simulink model "BanlanceCar"  (R2021b)
settings: Solver=FixedStepDiscrete  StartTime=0.0  StopTime=10.0  MaxStep=0.001  RelTol=1e-3
libraries: TIMERS_Lib x11, GPIO_Lib x7, USART_Lib x3, REG_Lib x2, STM32_Config_Lib x1
settings Model: Creator=Daniel  LastModifiedBy=Daniel
settings OptimizationCC: DefaultParameterBehavior=Inlined  EnhancedBackFolding=on  PassReuseOutputArgsAs=Individual arguments  ZeroExternalMemoryAtStartup=off  ZeroInternalMemoryAtStartup=off  OptimizeBlockOrder=speed  DifferentSizesBufferReuse=on  OptimizationCustomize=off  EfficientTunableParamExpr=on
settings DebuggingCC: ParameterTunabilityLossMsg=error
settings SFSimCC: SimCustomHeaderCode="#include \"myfile.h\""  SimUserSources="\"D:\\Simulink_stm32f4\\STM32F407VET6\\BalanceCar\\myfile.c\""  MATLABDynamicMemAlloc=off  CustomCodeUndefinedFunction=UseInterfaceOnly
settings RTWCC: Description=stm32 (Embedded Target)  SystemTargetFile=stm32.tlc  TemplateMakefile=stm32.tmf  GenerateReport=on
settings CodeAppCC: ForceParamTrailComments=on  IgnoreCustomStorageClasses=off  MaxIdLength=64  OperatorAnnotations=on  SimulinkDataObjDesc=on  SFDataObjDesc=on  CustomSymbolStrType=$N$R$M  StateflowObjectComments=on  MATLABSourceComments=on
settings STFCustomTargetCC: TargetLangStandard=C99 (ISO)  CodeReplacementLibrary=ARM CMSIS SIN COS  MultiwordLength=256  ParMdlRefBuildCompliant=on  IncludeMdlTerminateFcn=off  CombineOutputUpdateFcns=on  ERTCustomFileBanners=on  SupportContinuousTime=off  SupportNonInlinedSFcns=off  RemoveResetFunc=on  MATLABClassNameForMDSCustomization=Simulink.SoftwareTarget.ERTCustomization  GRTInterface=off  SystemTargetFile=stm32.tlc
settings ERTTargetCC: TargetLangStandard=C99 (ISO)  CodeReplacementLibrary=ARM CMSIS SIN COS  CompOptLevelCompliant=off  ConcurrentExecutionCompliant=off  IncludeMdlTerminateFcn=off  ModelStepFunctionPrototypeControlCompliant=off  CPPClassGenCompliant=off  UseToolchainInfoCompliant=off  ExtModeStaticAllocSize=256  ExtModeMexFile=ext_serial_win32_comm  ExtModeMexArgs=0,1,115200,10  InlinedParameterPlacement=NonHierarchical  ERTSrcFileBannerTemplate=sourceFileTemplate.cgt  ERTHdrFileBannerTemplate=sourceFileTemplate.cgt  ERTDataSrcFileTemplate=sourceFileTemplate.cgt  ERTDataHdrFileTemplate=sourceFileTemplate.cgt  ERTCustomFileTemplate=customRoutineProcess.tlc

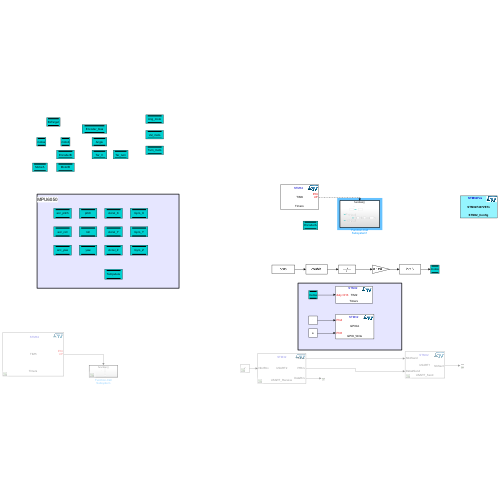
[thumbnail: Simulink's stored preview of the top-level diagram]
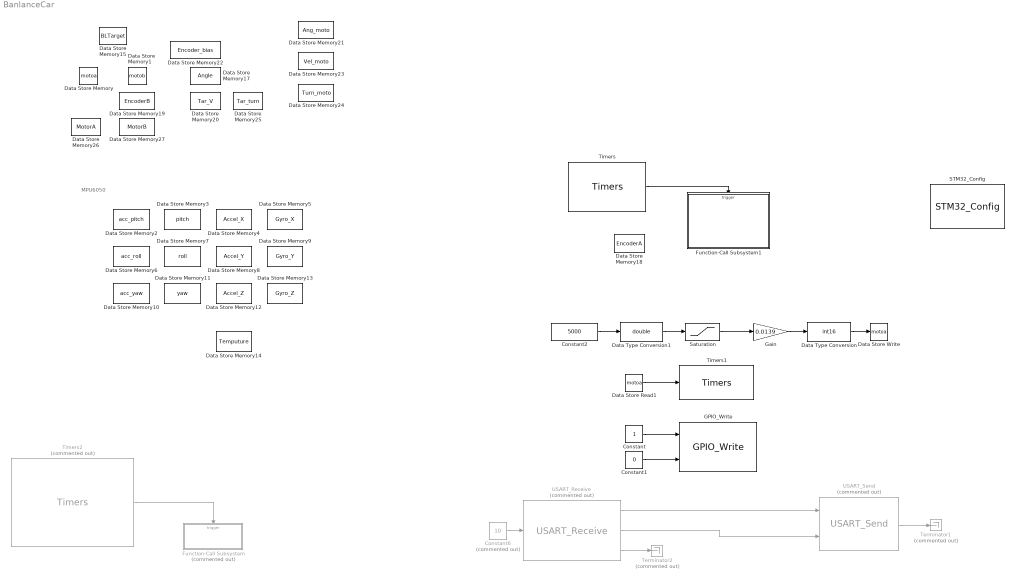
== system BanlanceCar ==
  note: MPU6050
  Constant : Constant
  Constant1 : Constant  Value=0
  Constant2 : Constant  Value=5000
  Constant6 : Constant  Commented=on  Value=10  OutDataTypeStr=uint16
  Data Store Memory : DataStoreMemory  DataStoreName=motoa  ReadBeforeWriteMsg=warning  WriteAfterWriteMsg=warning  WriteAfterReadMsg=warning  ShowAdditionalParam=off
  Data Store Memory1 : DataStoreMemory  DataStoreName=motob  ReadBeforeWriteMsg=warning  WriteAfterWriteMsg=warning  WriteAfterReadMsg=warning  ShowAdditionalParam=off
  Data Store Memory10 : DataStoreMemory  DataStoreName=acc_yaw  ReadBeforeWriteMsg=warning  WriteAfterWriteMsg=warning  WriteAfterReadMsg=warning  ShowAdditionalParam=off
  Data Store Memory11 : DataStoreMemory  DataStoreName=yaw  ReadBeforeWriteMsg=warning  WriteAfterWriteMsg=warning  WriteAfterReadMsg=warning  ShowAdditionalParam=off
  Data Store Memory12 : DataStoreMemory  DataStoreName=Accel_Z  ReadBeforeWriteMsg=warning  WriteAfterWriteMsg=warning  WriteAfterReadMsg=warning  ShowAdditionalParam=off
  Data Store Memory13 : DataStoreMemory  DataStoreName=Gyro_Z  ReadBeforeWriteMsg=warning  WriteAfterWriteMsg=warning  WriteAfterReadMsg=warning  ShowAdditionalParam=off
  Data Store Memory14 : DataStoreMemory  DataStoreName=Temputure  ReadBeforeWriteMsg=warning  WriteAfterWriteMsg=warning  WriteAfterReadMsg=warning  ShowAdditionalParam=off
  Data Store Memory15 : DataStoreMemory  DataStoreName=BLTarget  ReadBeforeWriteMsg=warning  WriteAfterWriteMsg=warning  WriteAfterReadMsg=warning  ShowAdditionalParam=off
  Data Store Memory17 : DataStoreMemory  DataStoreName=Angle  ReadBeforeWriteMsg=warning  WriteAfterWriteMsg=warning  WriteAfterReadMsg=warning  ShowAdditionalParam=off
  Data Store Memory18 : DataStoreMemory  DataStoreName=EncoderA  ReadBeforeWriteMsg=warning  WriteAfterWriteMsg=warning  WriteAfterReadMsg=warning  ShowAdditionalParam=off
  Data Store Memory19 : DataStoreMemory  DataStoreName=EncoderB  ReadBeforeWriteMsg=warning  WriteAfterWriteMsg=warning  WriteAfterReadMsg=warning  ShowAdditionalParam=off
  Data Store Memory2 : DataStoreMemory  DataStoreName=acc_pitch  ReadBeforeWriteMsg=warning  WriteAfterWriteMsg=warning  WriteAfterReadMsg=warning  ShowAdditionalParam=off
  Data Store Memory20 : DataStoreMemory  DataStoreName=Tar_V  ReadBeforeWriteMsg=warning  WriteAfterWriteMsg=warning  WriteAfterReadMsg=warning  ShowAdditionalParam=off
  Data Store Memory21 : DataStoreMemory  DataStoreName=Ang_moto  ReadBeforeWriteMsg=warning  WriteAfterWriteMsg=warning  WriteAfterReadMsg=warning  ShowAdditionalParam=off
  Data Store Memory22 : DataStoreMemory  DataStoreName=Encoder_bias  ReadBeforeWriteMsg=warning  WriteAfterWriteMsg=warning  WriteAfterReadMsg=warning  ShowAdditionalParam=off
  Data Store Memory23 : DataStoreMemory  DataStoreName=Vel_moto  ReadBeforeWriteMsg=warning  WriteAfterWriteMsg=warning  WriteAfterReadMsg=warning  ShowAdditionalParam=off
  Data Store Memory24 : DataStoreMemory  DataStoreName=Turn_moto  ReadBeforeWriteMsg=warning  WriteAfterWriteMsg=warning  WriteAfterReadMsg=warning  ShowAdditionalParam=off
  Data Store Memory25 : DataStoreMemory  DataStoreName=Tar_turn  ReadBeforeWriteMsg=warning  WriteAfterWriteMsg=warning  WriteAfterReadMsg=warning  ShowAdditionalParam=off
  Data Store Memory26 : DataStoreMemory  DataStoreName=MotorA  ReadBeforeWriteMsg=warning  WriteAfterWriteMsg=warning  WriteAfterReadMsg=warning  ShowAdditionalParam=off
  Data Store Memory27 : DataStoreMemory  DataStoreName=MotorB  ReadBeforeWriteMsg=warning  WriteAfterWriteMsg=warning  WriteAfterReadMsg=warning  ShowAdditionalParam=off
  Data Store Memory3 : DataStoreMemory  DataStoreName=pitch  ReadBeforeWriteMsg=warning  WriteAfterWriteMsg=warning  WriteAfterReadMsg=warning  ShowAdditionalParam=off
  Data Store Memory4 : DataStoreMemory  DataStoreName=Accel_X  ReadBeforeWriteMsg=warning  WriteAfterWriteMsg=warning  WriteAfterReadMsg=warning  ShowAdditionalParam=off
  Data Store Memory5 : DataStoreMemory  DataStoreName=Gyro_X  ReadBeforeWriteMsg=warning  WriteAfterWriteMsg=warning  WriteAfterReadMsg=warning  ShowAdditionalParam=off
  Data Store Memory6 : DataStoreMemory  DataStoreName=acc_roll  ReadBeforeWriteMsg=warning  WriteAfterWriteMsg=warning  WriteAfterReadMsg=warning  ShowAdditionalParam=off
  Data Store Memory7 : DataStoreMemory  DataStoreName=roll  ReadBeforeWriteMsg=warning  WriteAfterWriteMsg=warning  WriteAfterReadMsg=warning  ShowAdditionalParam=off
  Data Store Memory8 : DataStoreMemory  DataStoreName=Accel_Y  ReadBeforeWriteMsg=warning  WriteAfterWriteMsg=warning  WriteAfterReadMsg=warning  ShowAdditionalParam=off
  Data Store Memory9 : DataStoreMemory  DataStoreName=Gyro_Y  ReadBeforeWriteMsg=warning  WriteAfterWriteMsg=warning  WriteAfterReadMsg=warning  ShowAdditionalParam=off
  Data Store Read1 : DataStoreRead  DataStoreName=motoa  IndexOptions=Index vector (dialog)  Indices=1  OutputSizes=1
  Data Store Write : DataStoreWrite  DataStoreName=motoa  IndexOptions=Index vector (dialog)  Indices=1  OutputSizes=1
  Data Type Conversion : DataTypeConversion  OutDataTypeStr=int16
  Data Type Conversion1 : DataTypeConversion  OutDataTypeStr=double
  Function-Call Subsystem : Subsystem  Commented=on  TreatAsAtomicUnit=on
  Function-Call Subsystem1 : Subsystem  TreatAsAtomicUnit=on
  GPIO_Write : GPIO_Lib/GPIO_Write  Port_name=GPIOA  Pin0=off  Toggle_Pin0=off  Pin1=off  Toggle_Pin1=off  Pin2=off  Toggle_Pin2=off  Pin3=off  Toggle_Pin3=off  Pin4=on  Toggle_Pin4=off  Pin5=on  Toggle_Pin5=off  Pin6=off  Toggle_Pin6=off  Pin7=off  Toggle_Pin7=off  Pin8=off  Toggle_Pin8=off  Pin9=off  Toggle_Pin9=off  Pin10=off  Toggle_Pin10=off  Pin11=off  Toggle_Pin11=off  Pin12=off  Toggle_Pin12=off  Pin13=off  Toggle_Pin13=off  Pin14=off  Toggle_Pin14=off  Pin15=off  Toggle_Pin15=off  PinList="GPIOA4  5  6  7GPIOB9  10GPIOD1  2"
      settings: SourceProductName=Target Support Package - STM32 Adapter
  Gain : Gain  Gain=0.0139
  STM32_Config : STM32_Config_Lib/STM32_Config  Priority=0  Project_Path=.\  Config_File=BalanceCar.ioc  MCU_Name=STM32F407VETx
      settings: SourceProductName=Target Support Package - STM32 Adapter
  Saturation : Saturate  UpperLimit=7000  LowerLimit=-7000
  Terminator1 : Terminator  Commented=on
  Terminator2 : Terminator  Commented=on
  Timers : TIMERS_Lib/Timers  currentTIM=TIM9  TIM_Name=TIM9  sysUsingTimer=off  TIM_APBClock=72000000  TIM_Set_Clk=off  TIM_Prescaler=7199  TIM_Clock=10000.00  Variable_frequency=off  TIM_Set_OutFreq=off  TIM_ARR=10000  Output_frequency=1.00  Repetition_counter=0  TIM_Mode=Up  TIM_DMA=none  TIM_IRQ=on  TIM_IRQ_ONLY=on  TIM_UP=on  TIM_TRG=off  TIM_COM=off  TIM_BRK=off  NbTIM=5  CH1_enable=off  CH1N_enable=off  CH1_type=Unknown  CH1_DMA=off  CH1_int=off  CH1_edge=Rising  CH1_div=1  CH1_variable_duty=off  CH1_set_pulse=off  CH1_output_duty=0.00  CH1_pulse=0  CH2_enable=off  CH2N_enable=off  CH2_type=Unknown  CH2_DMA=off  CH2_int=off  CH2_edge=Rising  CH2_div=1  CH2_variable_duty=off  CH2_set_pulse=off  CH2_output_duty=0.00  CH2_pulse=0  CH3_enable=off  CH3N_enable=off  CH3_type=Unknown  CH3_DMA=off  CH3_int=off  CH3_edge=Rising  CH3_div=1  CH3_variable_duty=off  CH3_set_pulse=off  CH3_output_duty=0.00  CH3_pulse=0  CH4_enable=off  CH4N_enable=off  CH4_type=Unknown  CH4_DMA=off  CH4_int=off  CH4_edge=Rising  CH4_div=1  CH4_variable_duty=off  CH4_set_pulse=off  CH4_output_duty=0.00  CH4_pulse=0
      settings: SourceProductName=Target Support Package - STM32 Adapter
  Timers1 : TIMERS_Lib/Timers  currentTIM=TIM2  TIM_Name=TIM2  sysUsingTimer=off  TIM_APBClock=72000000  TIM_Set_Clk=off  TIM_Prescaler=0  TIM_Clock=72000000.00  Variable_frequency=off  TIM_Set_OutFreq=off  TIM_ARR=7199  Output_frequency=10001.39  Repetition_counter=0  TIM_Mode=Up  TIM_DMA=none  TIM_IRQ=on  TIM_IRQ_ONLY=off  TIM_UP=off  TIM_TRG=off  TIM_COM=off  TIM_BRK=off  NbTIM=5  CH1_enable=off  CH1N_enable=off  CH1_type=Unknown  CH1_DMA=off  CH1_int=off  CH1_edge=Rising  CH1_div=1  CH1_variable_duty=off  CH1_set_pulse=off  CH1_output_duty=0.00  CH1_pulse=0  CH2_enable=off  CH2N_enable=off  CH2_type=Unknown  CH2_DMA=off  CH2_int=off  CH2_edge=Rising  CH2_div=1  CH2_variable_duty=off  CH2_set_pulse=off  CH2_output_duty=0.00  CH2_pulse=0  CH3_enable=on  CH3N_enable=off  CH3_type=Output_PWM  CH3_DMA=off  CH3_int=off  CH3_edge=Rising  CH3_div=1  CH3_variable_duty=on  CH3_set_pulse=off  CH3_output_duty=6.93  CH3_pulse=500-1  CH4_enable=on  CH4N_enable=off  CH4_type=Output_PWM  CH4_DMA=off  CH4_int=off  CH4_edge=Rising  CH4_div=1  CH4_variable_duty=off  CH4_set_pulse=off  CH4_output_duty=0.00  CH4_pulse=0
      settings: SourceProductName=Target Support Package - STM32 Adapter
  Timers2 : TIMERS_Lib/Timers  Commented=on  currentTIM=TIM5  TIM_Name=TIM5  sysUsingTimer=off  TIM_APBClock=72000000  TIM_Set_Clk=off  TIM_Prescaler=7199  TIM_Clock=10000.00  Variable_frequency=off  TIM_Set_OutFreq=off  TIM_ARR=1  Output_frequency=10000.00  Repetition_counter=0  TIM_Mode=Up  TIM_DMA=none  TIM_IRQ=on  TIM_IRQ_ONLY=on  TIM_UP=on  TIM_TRG=off  TIM_COM=off  TIM_BRK=off  NbTIM=4  CH1_enable=off  CH1N_enable=off  CH1_type=Unknown  CH1_DMA=off  CH1_int=off  CH1_edge=Rising  CH1_div=1  CH1_variable_duty=off  CH1_set_pulse=off  CH1_output_duty=0.00  CH1_pulse=0  CH2_enable=off  CH2N_enable=off  CH2_type=Unknown  CH2_DMA=off  CH2_int=off  CH2_edge=Rising  CH2_div=1  CH2_variable_duty=off  CH2_set_pulse=off  CH2_output_duty=0.00  CH2_pulse=0  CH3_enable=off  CH3N_enable=off  CH3_type=Unknown  CH3_DMA=off  CH3_int=off  CH3_edge=Rising  CH3_div=1  CH3_variable_duty=off  CH3_set_pulse=off  CH3_output_duty=0.00  CH3_pulse=0  CH4_enable=off  CH4N_enable=off  CH4_type=Unknown  CH4_DMA=off  CH4_int=off  CH4_edge=Rising  CH4_div=1  CH4_variable_duty=off  CH4_set_pulse=off  CH4_output_duty=0.00  CH4_pulse=0
      settings: SourceProductName=Target Support Package - STM32 Adapter
  USART_Receive : USART_Lib/USART_Receive  Commented=on  USART_name=USART2  Buff_size=512  nbUsart=2  Soft_it=on  Soft_num=1  usartMode=Asynchronous  usartDma_Rx=off  usartDma_Tx=off  usartIt=on
      settings: SourceProductName=Target Support Package - STM32 Adapter
  USART_Send : USART_Lib/USART_Send  Commented=on  USART_name=USART1  Buff_size=512  nbUsart=2  usartMode=Asynchronous  usartDma_Rx=off  usartDma_Tx=off  usartIt=on
      settings: SourceProductName=Target Support Package - STM32 Adapter
  wires:
  USART_Receive/1 -> USART_Send/1
  Constant6/1 -> USART_Receive/1
  USART_Send/1 -> Terminator1/1
  USART_Receive/2 -> USART_Send/2
  USART_Receive/3 -> Terminator2/1
  Timers2/1 -> Function-Call Subsystem/Trigger
  Timers/1 -> Function-Call Subsystem1/Trigger
  Data Type Conversion1/1 -> Saturation/1
  Saturation/1 -> Gain/1
  Data Type Conversion/1 -> Data Store Write/1
  Gain/1 -> Data Type Conversion/1
  Constant1/1 -> GPIO_Write/2
  Constant/1 -> GPIO_Write/1
  Data Store Read1/1 -> Timers1/1
  Constant2/1 -> Data Type Conversion1/1

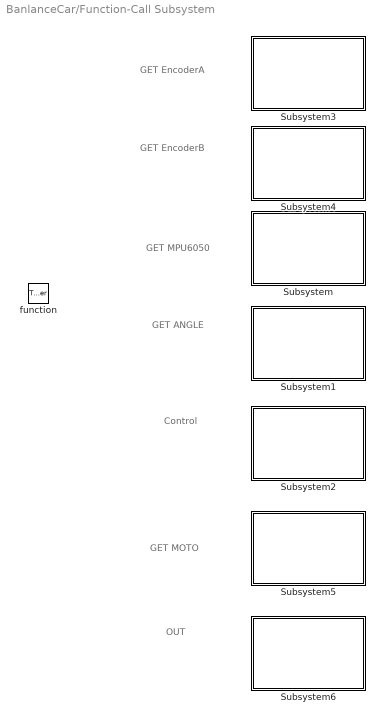
== system BanlanceCar/Function-Call Subsystem ==
  note: OUT
  note: GET MOTO
  note: GET EncoderB
  note: GET EncoderA
  note: Control
  note: GET ANGLE
  note: GET MPU6050
  function : TriggerPort  TriggerType=function-call  VariantControl=(inherit)
  Subsystem : Subsystem
  Subsystem1 : Subsystem
  Subsystem2 : Subsystem
  Subsystem3 : Subsystem
  Subsystem4 : Subsystem
  Subsystem5 : Subsystem
  Subsystem6 : Subsystem

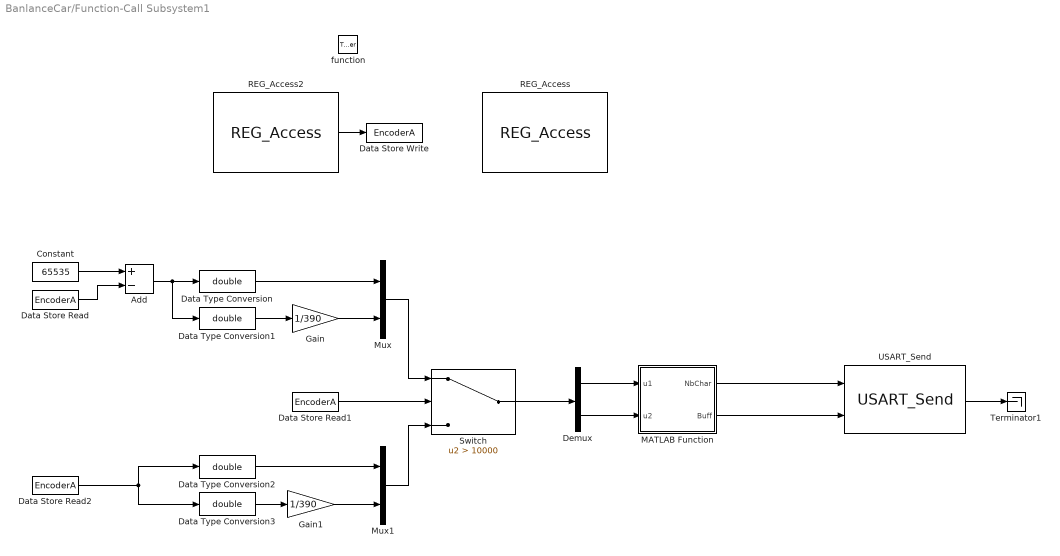
== system BanlanceCar/Function-Call Subsystem1 ==
  function : TriggerPort  TriggerType=function-call  VariantControl=(inherit)
  Add : Sum  Inputs=+-
  Constant : Constant  Value=65535
  Data Store Read : DataStoreRead  DataStoreName=EncoderA  IndexOptions=Index vector (dialog)  Indices=1  OutputSizes=1
  Data Store Read1 : DataStoreRead  DataStoreName=EncoderA  IndexOptions=Index vector (dialog)  Indices=1  OutputSizes=1
  Data Store Read2 : DataStoreRead  DataStoreName=EncoderA  IndexOptions=Index vector (dialog)  Indices=1  OutputSizes=1
  Data Store Write : DataStoreWrite  DataStoreName=EncoderA  IndexOptions=Index vector (dialog)  Indices=1  OutputSizes=1
  Data Type Conversion{,1..3} (4 alike) : DataTypeConversion  OutDataTypeStr=double
  Demux : Demux  Outputs=2
  Gain : Gain  Gain=1/390
  Gain1 : Gain  Gain=1/390
  MATLAB Function : MATLAB Function  TreatAsAtomicUnit=on
  Mux : Mux  Inputs=2
  Mux1 : Mux  Inputs=2
  REG_Access : REG_Lib/REG_Access  Peripheral=TIM1  RegName=CNT  RegRead=off  RegWrite=on  RegValueIn=off  RegValue=0  RegEqual=on  RegAnd=off  RegOr=off  RegComplement=off  currentPeriph=TIM1
      settings: SourceProductName=Target Support Package - STM32 Adapter
  REG_Access2 : REG_Lib/REG_Access  Priority=1  Peripheral=TIM1  RegName=CNT  RegRead=on  RegWrite=off  RegValueIn=off  RegValue=0  RegEqual=on  RegAnd=off  RegOr=off  RegComplement=off  currentPeriph=TIM1
      settings: SourceProductName=Target Support Package - STM32 Adapter
  Switch : Switch  Criteria=u2 > Threshold  Threshold=10000
  Terminator1 : Terminator
  USART_Send : USART_Lib/USART_Send  USART_name=USART1  Buff_size=512  nbUsart=2  usartMode=Asynchronous  usartDma_Rx=off  usartDma_Tx=off  usartIt=on
      settings: SourceProductName=Target Support Package - STM32 Adapter
  wires:
  REG_Access2/1 -> Data Store Write/1
  Data Store Read/1 -> Add/2
  Constant/1 -> Add/1
  Add/1 -> Data Type Conversion1/1, Data Type Conversion/1
  Data Type Conversion1/1 -> Gain/1
  Data Type Conversion/1 -> Mux/1
  Gain/1 -> Mux/2
  Data Store Read2/1 -> Data Type Conversion3/1, Data Type Conversion2/1
  Data Type Conversion3/1 -> Gain1/1
  Data Type Conversion2/1 -> Mux1/1
  Gain1/1 -> Mux1/2
  Mux/1 -> Switch/1
  Data Store Read1/1 -> Switch/2
  Mux1/1 -> Switch/3
  Switch/1 -> Demux/1
  Demux/1 -> MATLAB Function/1(u1)
  Demux/2 -> MATLAB Function/2(u2)
  MATLAB Function/1(NbChar) -> USART_Send/1
  MATLAB Function/2(Buff) -> USART_Send/2
  USART_Send/1 -> Terminator1/1

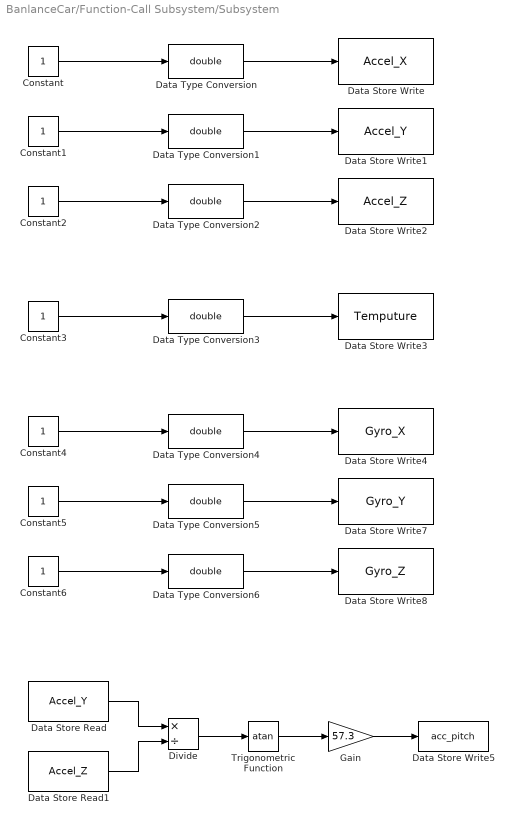
== system BanlanceCar/Function-Call Subsystem/Subsystem ==
  Constant{,1..6} (7 alike) : Constant
  Data Store Read : DataStoreRead  DataStoreName=Accel_Y  IndexOptions=Index vector (dialog)  Indices=1  OutputSizes=1
  Data Store Read1 : DataStoreRead  DataStoreName=Accel_Z  IndexOptions=Index vector (dialog)  Indices=1  OutputSizes=1
  Data Store Write : DataStoreWrite  DataStoreName=Accel_X  IndexOptions=Index vector (dialog)  Indices=1  OutputSizes=1
  Data Store Write1 : DataStoreWrite  DataStoreName=Accel_Y  IndexOptions=Index vector (dialog)  Indices=1  OutputSizes=1
  Data Store Write2 : DataStoreWrite  DataStoreName=Accel_Z  IndexOptions=Index vector (dialog)  Indices=1  OutputSizes=1
  Data Store Write3 : DataStoreWrite  DataStoreName=Temputure  IndexOptions=Index vector (dialog)  Indices=1  OutputSizes=1
  Data Store Write4 : DataStoreWrite  DataStoreName=Gyro_X  IndexOptions=Index vector (dialog)  Indices=1  OutputSizes=1
  Data Store Write5 : DataStoreWrite  DataStoreName=acc_pitch  IndexOptions=Index vector (dialog)  Indices=1  OutputSizes=1
  Data Store Write7 : DataStoreWrite  DataStoreName=Gyro_Y  IndexOptions=Index vector (dialog)  Indices=1  OutputSizes=1
  Data Store Write8 : DataStoreWrite  DataStoreName=Gyro_Z  IndexOptions=Index vector (dialog)  Indices=1  OutputSizes=1
  Data Type Conversion{,1..6} (7 alike) : DataTypeConversion  OutDataTypeStr=double
  Divide : Product  Inputs=*/
  Gain : Gain  Gain=57.3
  Trigonometric Function : Trigonometry  Operator=atan
  wires:
  Data Type Conversion/1 -> Data Store Write/1
  Data Type Conversion2/1 -> Data Store Write2/1
  Data Type Conversion1/1 -> Data Store Write1/1
  Data Type Conversion6/1 -> Data Store Write8/1
  Data Type Conversion5/1 -> Data Store Write7/1
  Data Type Conversion4/1 -> Data Store Write4/1
  Data Type Conversion3/1 -> Data Store Write3/1
  Constant/1 -> Data Type Conversion/1
  Constant1/1 -> Data Type Conversion1/1
  Constant2/1 -> Data Type Conversion2/1
  Constant3/1 -> Data Type Conversion3/1
  Constant4/1 -> Data Type Conversion4/1
  Constant5/1 -> Data Type Conversion5/1
  Constant6/1 -> Data Type Conversion6/1
  Data Store Read/1 -> Divide/1
  Data Store Read1/1 -> Divide/2
  Divide/1 -> Trigonometric Function/1
  Trigonometric Function/1 -> Gain/1
  Gain/1 -> Data Store Write5/1

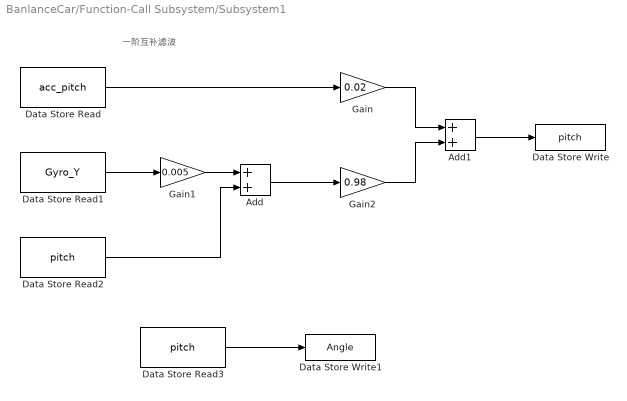
== system BanlanceCar/Function-Call Subsystem/Subsystem1 ==
  note: 一阶互补滤波
  Add : Sum
  Add1 : Sum
  Data Store Read : DataStoreRead  DataStoreName=acc_pitch  IndexOptions=Index vector (dialog)  Indices=1  OutputSizes=1
  Data Store Read1 : DataStoreRead  DataStoreName=Gyro_Y  IndexOptions=Index vector (dialog)  Indices=1  OutputSizes=1
  Data Store Read2 : DataStoreRead  DataStoreName=pitch  IndexOptions=Index vector (dialog)  Indices=1  OutputSizes=1
  Data Store Read3 : DataStoreRead  DataStoreName=pitch  IndexOptions=Index vector (dialog)  Indices=1  OutputSizes=1
  Data Store Write : DataStoreWrite  DataStoreName=pitch  IndexOptions=Index vector (dialog)  Indices=1  OutputSizes=1
  Data Store Write1 : DataStoreWrite  DataStoreName=Angle  IndexOptions=Index vector (dialog)  Indices=1  OutputSizes=1
  Gain : Gain  Gain=0.02
  Gain1 : Gain  Gain=0.005
  Gain2 : Gain  Gain=0.98
  wires:
  Data Store Read/1 -> Gain/1
  Data Store Read1/1 -> Gain1/1
  Data Store Read2/1 -> Add/2
  Gain1/1 -> Add/1
  Add/1 -> Gain2/1
  Gain/1 -> Add1/1
  Gain2/1 -> Add1/2
  Add1/1 -> Data Store Write/1
  Data Store Read3/1 -> Data Store Write1/1

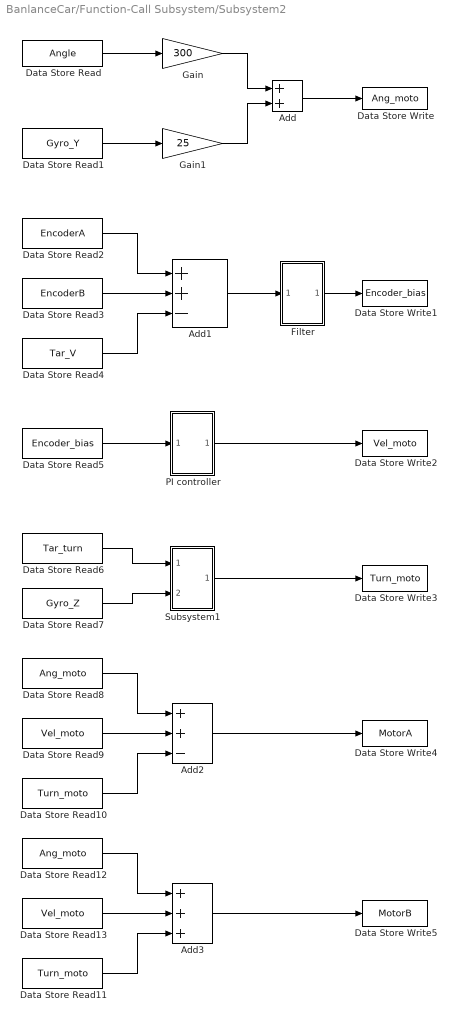
== system BanlanceCar/Function-Call Subsystem/Subsystem2 ==
  Add : Sum
  Add1 : Sum  Inputs=++-
  Add2 : Sum  Priority=5  Inputs=++-
  Add3 : Sum  Priority=5  Inputs=+++
  Data Store Read : DataStoreRead  DataStoreName=Angle  IndexOptions=Index vector (dialog)  Indices=1  OutputSizes=1
  Data Store Read1 : DataStoreRead  DataStoreName=Gyro_Y  IndexOptions=Index vector (dialog)  Indices=1  OutputSizes=1
  Data Store Read10 : DataStoreRead  DataStoreName=Turn_moto  IndexOptions=Index vector (dialog)  Indices=1  OutputSizes=1
  Data Store Read11 : DataStoreRead  DataStoreName=Turn_moto  IndexOptions=Index vector (dialog)  Indices=1  OutputSizes=1
  Data Store Read12 : DataStoreRead  DataStoreName=Ang_moto  IndexOptions=Index vector (dialog)  Indices=1  OutputSizes=1
  Data Store Read13 : DataStoreRead  DataStoreName=Vel_moto  IndexOptions=Index vector (dialog)  Indices=1  OutputSizes=1
  Data Store Read2 : DataStoreRead  DataStoreName=EncoderA  IndexOptions=Index vector (dialog)  Indices=1  OutputSizes=1
  Data Store Read3 : DataStoreRead  DataStoreName=EncoderB  IndexOptions=Index vector (dialog)  Indices=1  OutputSizes=1
  Data Store Read4 : DataStoreRead  DataStoreName=Tar_V  IndexOptions=Index vector (dialog)  Indices=1  OutputSizes=1
  Data Store Read5 : DataStoreRead  DataStoreName=Encoder_bias  IndexOptions=Index vector (dialog)  Indices=1  OutputSizes=1
  Data Store Read6 : DataStoreRead  DataStoreName=Tar_turn  IndexOptions=Index vector (dialog)  Indices=1  OutputSizes=1
  Data Store Read7 : DataStoreRead  DataStoreName=Gyro_Z  IndexOptions=Index vector (dialog)  Indices=1  OutputSizes=1
  Data Store Read8 : DataStoreRead  DataStoreName=Ang_moto  IndexOptions=Index vector (dialog)  Indices=1  OutputSizes=1
  Data Store Read9 : DataStoreRead  DataStoreName=Vel_moto  IndexOptions=Index vector (dialog)  Indices=1  OutputSizes=1
  Data Store Write : DataStoreWrite  DataStoreName=Ang_moto  IndexOptions=Index vector (dialog)  Indices=1  OutputSizes=1
  Data Store Write1 : DataStoreWrite  DataStoreName=Encoder_bias  IndexOptions=Index vector (dialog)  Indices=1  OutputSizes=1
  Data Store Write2 : DataStoreWrite  DataStoreName=Vel_moto  IndexOptions=Index vector (dialog)  Indices=1  OutputSizes=1
  Data Store Write3 : DataStoreWrite  DataStoreName=Turn_moto  IndexOptions=Index vector (dialog)  Indices=1  OutputSizes=1
  Data Store Write4 : DataStoreWrite  DataStoreName=MotorA  IndexOptions=Index vector (dialog)  Indices=1  OutputSizes=1
  Data Store Write5 : DataStoreWrite  DataStoreName=MotorB  IndexOptions=Index vector (dialog)  Indices=1  OutputSizes=1
  Filter : Subsystem
  Gain : Gain  Gain=300
  Gain1 : Gain  Gain=25
  PI controller : Subsystem  Priority=3
  Subsystem1 : Subsystem  Priority=4
  wires:
  Data Store Read/1 -> Gain/1
  Data Store Read1/1 -> Gain1/1
  Gain/1 -> Add/1
  Gain1/1 -> Add/2
  Add/1 -> Data Store Write/1
  Data Store Read2/1 -> Add1/1
  Data Store Read3/1 -> Add1/2
  Data Store Read4/1 -> Add1/3
  Add1/1 -> Filter/1(In1)
  Filter/1(Out1) -> Data Store Write1/1
  Data Store Read5/1 -> PI controller/1(In1)
  PI controller/1(Out1) -> Data Store Write2/1
  Data Store Read6/1 -> Subsystem1/1(In1)
  Data Store Read7/1 -> Subsystem1/2(In2)
  Subsystem1/1(Out1) -> Data Store Write3/1
  Data Store Read8/1 -> Add2/1
  Data Store Read9/1 -> Add2/2
  Data Store Read10/1 -> Add2/3
  Add2/1 -> Data Store Write4/1
  Add3/1 -> Data Store Write5/1
  Data Store Read11/1 -> Add3/3
  Data Store Read13/1 -> Add3/2
  Data Store Read12/1 -> Add3/1

== system BanlanceCar/Function-Call Subsystem/Subsystem3 ==
  Timers : TIMERS_Lib/Timers  currentTIM=TIM1  TIM_Name=TIM1  sysUsingTimer=off  TIM_APBClock=72000000  TIM_Set_Clk=off  TIM_Prescaler=0  TIM_Clock=72000000.00  Variable_frequency=off  TIM_Set_OutFreq=off  TIM_ARR=65536  Output_frequency=1098.63  Repetition_counter=0  TIM_Mode=Up  TIM_DMA=none  TIM_IRQ=off  TIM_IRQ_ONLY=on  TIM_UP=off  TIM_TRG=off  TIM_COM=off  TIM_BRK=off  NbTIM=4  CH1_enable=on  CH1N_enable=on  CH1_type=Unknown  CH1_DMA=off  CH1_int=off  CH1_edge=Rising  CH1_div=1  CH1_variable_duty=off  CH1_set_pulse=off  CH1_output_duty=0.00  CH1_pulse=0  CH2_enable=on  CH2N_enable=off  CH2_type=Unknown  CH2_DMA=off  CH2_int=off  CH2_edge=Rising  CH2_div=1  CH2_variable_duty=off  CH2_set_pulse=off  CH2_output_duty=0.00  CH2_pulse=0  CH3_enable=off  CH3N_enable=off  CH3_type=Unknown  CH3_DMA=off  CH3_int=off  CH3_edge=Rising  CH3_div=1  CH3_variable_duty=off  CH3_set_pulse=off  CH3_output_duty=0.00  CH3_pulse=0  CH4_enable=off  CH4N_enable=off  CH4_type=Unknown  CH4_DMA=off  CH4_int=off  CH4_edge=Rising  CH4_div=1  CH4_variable_duty=off  CH4_set_pulse=off  CH4_output_duty=0.00  CH4_pulse=0
      settings: SourceProductName=Target Support Package - STM32 Adapter

== system BanlanceCar/Function-Call Subsystem/Subsystem4 ==
  Timers : TIMERS_Lib/Timers  currentTIM=TIM4  TIM_Name=TIM4  sysUsingTimer=off  TIM_APBClock=72000000  TIM_Set_Clk=off  TIM_Prescaler=0  TIM_Clock=72000000.00  Variable_frequency=off  TIM_Set_OutFreq=off  TIM_ARR=1  Output_frequency=72000000.00  Repetition_counter=0  TIM_Mode=Up  TIM_DMA=none  TIM_IRQ=on  TIM_IRQ_ONLY=on  TIM_UP=off  TIM_TRG=off  TIM_COM=off  TIM_BRK=off  NbTIM=4  CH1_enable=on  CH1N_enable=off  CH1_type=Unknown  CH1_DMA=off  CH1_int=off  CH1_edge=Rising  CH1_div=1  CH1_variable_duty=off  CH1_set_pulse=off  CH1_output_duty=0.00  CH1_pulse=0  CH2_enable=on  CH2N_enable=off  CH2_type=Unknown  CH2_DMA=off  CH2_int=off  CH2_edge=Rising  CH2_div=1  CH2_variable_duty=off  CH2_set_pulse=off  CH2_output_duty=0.00  CH2_pulse=0  CH3_enable=off  CH3N_enable=off  CH3_type=Unknown  CH3_DMA=off  CH3_int=off  CH3_edge=Rising  CH3_div=1  CH3_variable_duty=off  CH3_set_pulse=off  CH3_output_duty=0.00  CH3_pulse=0  CH4_enable=off  CH4N_enable=off  CH4_type=Unknown  CH4_DMA=off  CH4_int=off  CH4_edge=Rising  CH4_div=1  CH4_variable_duty=off  CH4_set_pulse=off  CH4_output_duty=0.00  CH4_pulse=0
      settings: SourceProductName=Target Support Package - STM32 Adapter

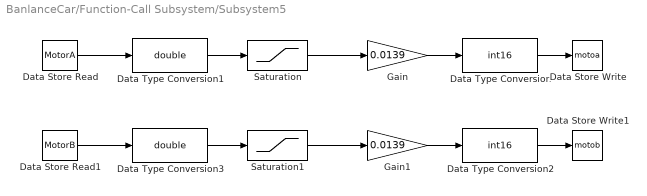
== system BanlanceCar/Function-Call Subsystem/Subsystem5 ==
  Data Store Read : DataStoreRead  DataStoreName=MotorA  IndexOptions=Index vector (dialog)  Indices=1  OutputSizes=1
  Data Store Read1 : DataStoreRead  DataStoreName=MotorB  IndexOptions=Index vector (dialog)  Indices=1  OutputSizes=1
  Data Store Write : DataStoreWrite  DataStoreName=motoa  IndexOptions=Index vector (dialog)  Indices=1  OutputSizes=1
  Data Store Write1 : DataStoreWrite  DataStoreName=motob  IndexOptions=Index vector (dialog)  Indices=1  OutputSizes=1
  Data Type Conversion : DataTypeConversion  OutDataTypeStr=int16
  Data Type Conversion1 : DataTypeConversion  OutDataTypeStr=double
  Data Type Conversion2 : DataTypeConversion  OutDataTypeStr=int16
  Data Type Conversion3 : DataTypeConversion  OutDataTypeStr=double
  Gain : Gain  Gain=0.0139
  Gain1 : Gain  Gain=0.0139
  Saturation : Saturate  UpperLimit=7000  LowerLimit=-7000
  Saturation1 : Saturate  UpperLimit=7000  LowerLimit=-7000
  wires:
  Data Type Conversion3/1 -> Saturation1/1
  Data Type Conversion/1 -> Data Store Write/1
  Data Type Conversion2/1 -> Data Store Write1/1
  Saturation1/1 -> Gain1/1
  Data Type Conversion1/1 -> Saturation/1
  Gain/1 -> Data Type Conversion/1
  Gain1/1 -> Data Type Conversion2/1
  Data Store Read/1 -> Data Type Conversion1/1
  Data Store Read1/1 -> Data Type Conversion3/1
  Saturation/1 -> Gain/1

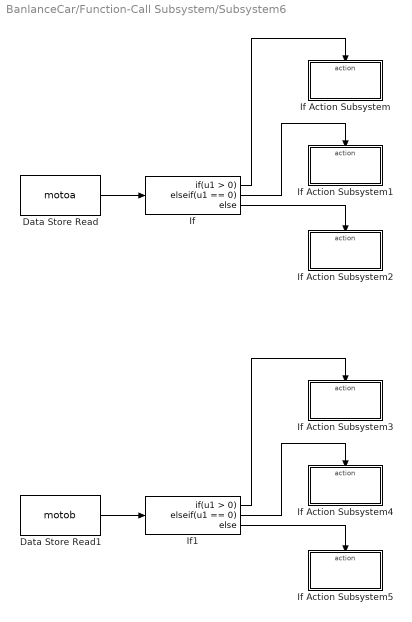
== system BanlanceCar/Function-Call Subsystem/Subsystem6 ==
  Data Store Read : DataStoreRead  DataStoreName=motoa  IndexOptions=Index vector (dialog)  Indices=1  OutputSizes=1
  Data Store Read1 : DataStoreRead  DataStoreName=motob  IndexOptions=Index vector (dialog)  Indices=1  OutputSizes=1
  If : If  ElseIfExpressions=u1 == 0
  If Action Subsystem : Subsystem  TreatAsAtomicUnit=on
  If Action Subsystem1 : Subsystem  TreatAsAtomicUnit=on
  If Action Subsystem2 : Subsystem  TreatAsAtomicUnit=on
  If Action Subsystem3 : Subsystem  TreatAsAtomicUnit=on
  If Action Subsystem4 : Subsystem  TreatAsAtomicUnit=on
  If Action Subsystem5 : Subsystem  TreatAsAtomicUnit=on
  If1 : If  ElseIfExpressions=u1 == 0
  wires:
  Data Store Read/1 -> If/1
  If/1 -> If Action Subsystem/Action
  If/2 -> If Action Subsystem1/Action
  If/3 -> If Action Subsystem2/Action
  If1/3 -> If Action Subsystem5/Action
  If1/2 -> If Action Subsystem4/Action
  If1/1 -> If Action Subsystem3/Action
  Data Store Read1/1 -> If1/1

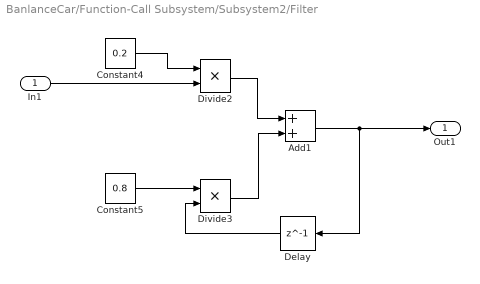
== system BanlanceCar/Function-Call Subsystem/Subsystem2/Filter ==
  In1 : Inport
  Add1 : Sum
  Constant4 : Constant  Value=0.2
  Constant5 : Constant  Value=0.8
  Delay : Delay  DelayLength=1  InitialCondition=0
  Divide2 : Product  Inputs=**
  Divide3 : Product  Inputs=**
  Out1 : Outport  VectorParamsAs1DForOutWhenUnconnected=off
  wires:
  Add1/1 -> Delay/1, Out1/1
  Constant5/1 -> Divide3/1
  In1/1 -> Divide2/2
  Divide3/1 -> Add1/2
  Delay/1 -> Divide3/2
  Constant4/1 -> Divide2/1
  Divide2/1 -> Add1/1

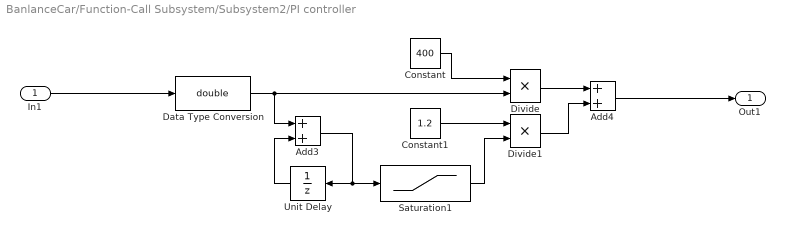
== system BanlanceCar/Function-Call Subsystem/Subsystem2/PI controller ==
  In1 : Inport
  Add3 : Sum  Priority=2
  Add4 : Sum  Priority=2
  Constant : Constant  Value=400  OutDataTypeStr=double
  Constant1 : Constant  Value=1.2  OutDataTypeStr=double
  Data Type Conversion : DataTypeConversion  OutDataTypeStr=double
  Divide : Product  Inputs=**
  Divide1 : Product  Inputs=**
  Saturation1 : Saturate  UpperLimit=10000  LowerLimit=-10000
  Unit Delay : UnitDelay  SampleTime=-1  HasFrameUpgradeWarning=on
  Out1 : Outport  VectorParamsAs1DForOutWhenUnconnected=off
  wires:
  Constant/1 -> Divide/1
  Unit Delay/1 -> Add3/2
  Add4/1 -> Out1/1
  Divide/1 -> Add4/1
  Data Type Conversion/1 -> Divide/2, Add3/1
  Divide1/1 -> Add4/2
  Constant1/1 -> Divide1/1
  Add3/1 -> Unit Delay/1, Saturation1/1
  In1/1 -> Data Type Conversion/1
  Saturation1/1 -> Divide1/2

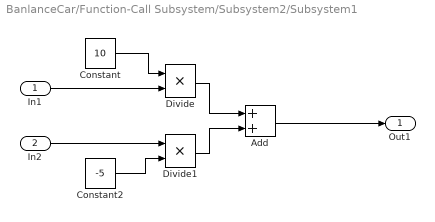
== system BanlanceCar/Function-Call Subsystem/Subsystem2/Subsystem1 ==
  In1 : Inport
  In2 : Inport  Port=2
  Add : Sum
  Constant : Constant  Value=10
  Constant2 : Constant  Value=-5
  Divide : Product  Inputs=**
  Divide1 : Product  Inputs=**
  Out1 : Outport  VectorParamsAs1DForOutWhenUnconnected=off
  wires:
  In2/1 -> Divide1/1
  In1/1 -> Divide/2
  Divide/1 -> Add/1
  Add/1 -> Out1/1
  Constant2/1 -> Divide1/2
  Constant/1 -> Divide/1
  Divide1/1 -> Add/2

== system BanlanceCar/Function-Call Subsystem/Subsystem6/If Action Subsystem ==
  Action Port : ActionPort  ActionPortLabel=if(u1 > 0)
  Constant : Constant
  Constant1 : Constant  Value=0
  Data Store Read : DataStoreRead  DataStoreName=motoa  IndexOptions=Index vector (dialog)  Indices=1  OutputSizes=1
  GPIO_Write : GPIO_Lib/GPIO_Write  Port_name=GPIOA  Pin0=off  Toggle_Pin0=off  Pin1=off  Toggle_Pin1=off  Pin2=off  Toggle_Pin2=off  Pin3=off  Toggle_Pin3=off  Pin4=on  Toggle_Pin4=off  Pin5=on  Toggle_Pin5=off  Pin6=off  Toggle_Pin6=off  Pin7=off  Toggle_Pin7=off  Pin8=off  Toggle_Pin8=off  Pin9=off  Toggle_Pin9=off  Pin10=off  Toggle_Pin10=off  Pin11=off  Toggle_Pin11=off  Pin12=off  Toggle_Pin12=off  Pin13=off  Toggle_Pin13=off  Pin14=off  Toggle_Pin14=off  Pin15=off  Toggle_Pin15=off  PinList="GPIOA4  5  6  7GPIOB9  10GPIOD1  2"
      settings: SourceProductName=Target Support Package - STM32 Adapter
  Timers : TIMERS_Lib/Timers  currentTIM=TIM2  TIM_Name=TIM2  sysUsingTimer=off  TIM_APBClock=72000000  TIM_Set_Clk=off  TIM_Prescaler=0  TIM_Clock=72000000.00  Variable_frequency=off  TIM_Set_OutFreq=off  TIM_ARR=7199  Output_frequency=10001.39  Repetition_counter=0  TIM_Mode=Up  TIM_DMA=none  TIM_IRQ=on  TIM_IRQ_ONLY=off  TIM_UP=off  TIM_TRG=off  TIM_COM=off  TIM_BRK=off  NbTIM=4  CH1_enable=off  CH1N_enable=off  CH1_type=Unknown  CH1_DMA=off  CH1_int=off  CH1_edge=Rising  CH1_div=1  CH1_variable_duty=off  CH1_set_pulse=off  CH1_output_duty=0.00  CH1_pulse=0  CH2_enable=off  CH2N_enable=off  CH2_type=Unknown  CH2_DMA=off  CH2_int=off  CH2_edge=Rising  CH2_div=1  CH2_variable_duty=off  CH2_set_pulse=off  CH2_output_duty=0.00  CH2_pulse=0  CH3_enable=on  CH3N_enable=off  CH3_type=Output_PWM  CH3_DMA=off  CH3_int=off  CH3_edge=Rising  CH3_div=1  CH3_variable_duty=on  CH3_set_pulse=off  CH3_output_duty=6.93  CH3_pulse=500-1  CH4_enable=on  CH4N_enable=off  CH4_type=Output_PWM  CH4_DMA=off  CH4_int=off  CH4_edge=Rising  CH4_div=1  CH4_variable_duty=off  CH4_set_pulse=off  CH4_output_duty=0.00  CH4_pulse=0
      settings: SourceProductName=Target Support Package - STM32 Adapter
  wires:
  Data Store Read/1 -> Timers/1
  Constant/1 -> GPIO_Write/1
  Constant1/1 -> GPIO_Write/2

== system BanlanceCar/Function-Call Subsystem/Subsystem6/If Action Subsystem1 ==
  Action Port : ActionPort  ActionPortLabel=elseif(u1 == 0)
  Constant : Constant  Value=0
  Constant1 : Constant  Value=0
  Data Store Read : DataStoreRead  DataStoreName=motoa  IndexOptions=Index vector (dialog)  Indices=1  OutputSizes=1
  GPIO_Write : GPIO_Lib/GPIO_Write  Port_name=GPIOA  Pin0=off  Toggle_Pin0=off  Pin1=off  Toggle_Pin1=off  Pin2=off  Toggle_Pin2=off  Pin3=off  Toggle_Pin3=off  Pin4=on  Toggle_Pin4=off  Pin5=on  Toggle_Pin5=off  Pin6=off  Toggle_Pin6=off  Pin7=off  Toggle_Pin7=off  Pin8=off  Toggle_Pin8=off  Pin9=off  Toggle_Pin9=off  Pin10=off  Toggle_Pin10=off  Pin11=off  Toggle_Pin11=off  Pin12=off  Toggle_Pin12=off  Pin13=off  Toggle_Pin13=off  Pin14=off  Toggle_Pin14=off  Pin15=off  Toggle_Pin15=off  PinList="GPIOA4  5  6  7GPIOB9  10GPIOD1  2"
      settings: SourceProductName=Target Support Package - STM32 Adapter
  Timers : TIMERS_Lib/Timers  currentTIM=TIM2  TIM_Name=TIM2  sysUsingTimer=off  TIM_APBClock=72000000  TIM_Set_Clk=off  TIM_Prescaler=0  TIM_Clock=72000000.00  Variable_frequency=off  TIM_Set_OutFreq=off  TIM_ARR=7199  Output_frequency=10001.39  Repetition_counter=0  TIM_Mode=Up  TIM_DMA=none  TIM_IRQ=on  TIM_IRQ_ONLY=off  TIM_UP=off  TIM_TRG=off  TIM_COM=off  TIM_BRK=off  NbTIM=4  CH1_enable=off  CH1N_enable=off  CH1_type=Unknown  CH1_DMA=off  CH1_int=off  CH1_edge=Rising  CH1_div=1  CH1_variable_duty=off  CH1_set_pulse=off  CH1_output_duty=0.00  CH1_pulse=0  CH2_enable=off  CH2N_enable=off  CH2_type=Unknown  CH2_DMA=off  CH2_int=off  CH2_edge=Rising  CH2_div=1  CH2_variable_duty=off  CH2_set_pulse=off  CH2_output_duty=0.00  CH2_pulse=0  CH3_enable=on  CH3N_enable=off  CH3_type=Output_PWM  CH3_DMA=off  CH3_int=off  CH3_edge=Rising  CH3_div=1  CH3_variable_duty=on  CH3_set_pulse=off  CH3_output_duty=6.93  CH3_pulse=500-1  CH4_enable=on  CH4N_enable=off  CH4_type=Output_PWM  CH4_DMA=off  CH4_int=off  CH4_edge=Rising  CH4_div=1  CH4_variable_duty=off  CH4_set_pulse=off  CH4_output_duty=0.00  CH4_pulse=0
      settings: SourceProductName=Target Support Package - STM32 Adapter
  wires:
  Constant1/1 -> GPIO_Write/2
  Constant/1 -> GPIO_Write/1
  Data Store Read/1 -> Timers/1

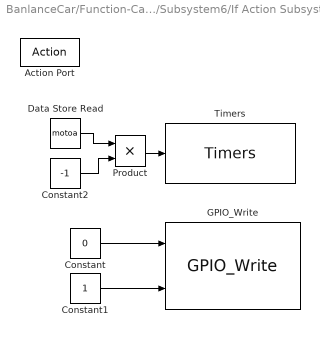
== system BanlanceCar/Function-Call Subsystem/Subsystem6/If Action Subsystem2 ==
  Action Port : ActionPort  ActionPortLabel=else
  Constant : Constant  Value=0
  Constant1 : Constant
  Constant2 : Constant  Value=-1
  Data Store Read : DataStoreRead  DataStoreName=motoa  IndexOptions=Index vector (dialog)  Indices=1  OutputSizes=1
  GPIO_Write : GPIO_Lib/GPIO_Write  Port_name=GPIOA  Pin0=off  Toggle_Pin0=off  Pin1=off  Toggle_Pin1=off  Pin2=off  Toggle_Pin2=off  Pin3=off  Toggle_Pin3=off  Pin4=on  Toggle_Pin4=off  Pin5=on  Toggle_Pin5=off  Pin6=off  Toggle_Pin6=off  Pin7=off  Toggle_Pin7=off  Pin8=off  Toggle_Pin8=off  Pin9=off  Toggle_Pin9=off  Pin10=off  Toggle_Pin10=off  Pin11=off  Toggle_Pin11=off  Pin12=off  Toggle_Pin12=off  Pin13=off  Toggle_Pin13=off  Pin14=off  Toggle_Pin14=off  Pin15=off  Toggle_Pin15=off  PinList="GPIOA4  5  6  7GPIOB9  10GPIOD1  2"
      settings: SourceProductName=Target Support Package - STM32 Adapter
  Product : Product
  Timers : TIMERS_Lib/Timers  currentTIM=TIM2  TIM_Name=TIM2  sysUsingTimer=off  TIM_APBClock=72000000  TIM_Set_Clk=off  TIM_Prescaler=0  TIM_Clock=72000000.00  Variable_frequency=off  TIM_Set_OutFreq=off  TIM_ARR=7199  Output_frequency=10001.39  Repetition_counter=0  TIM_Mode=Up  TIM_DMA=none  TIM_IRQ=on  TIM_IRQ_ONLY=off  TIM_UP=off  TIM_TRG=off  TIM_COM=off  TIM_BRK=off  NbTIM=4  CH1_enable=off  CH1N_enable=off  CH1_type=Unknown  CH1_DMA=off  CH1_int=off  CH1_edge=Rising  CH1_div=1  CH1_variable_duty=off  CH1_set_pulse=off  CH1_output_duty=0.00  CH1_pulse=0  CH2_enable=off  CH2N_enable=off  CH2_type=Unknown  CH2_DMA=off  CH2_int=off  CH2_edge=Rising  CH2_div=1  CH2_variable_duty=off  CH2_set_pulse=off  CH2_output_duty=0.00  CH2_pulse=0  CH3_enable=on  CH3N_enable=off  CH3_type=Output_PWM  CH3_DMA=off  CH3_int=off  CH3_edge=Rising  CH3_div=1  CH3_variable_duty=on  CH3_set_pulse=off  CH3_output_duty=6.93  CH3_pulse=500-1  CH4_enable=on  CH4N_enable=off  CH4_type=Output_PWM  CH4_DMA=off  CH4_int=off  CH4_edge=Rising  CH4_div=1  CH4_variable_duty=off  CH4_set_pulse=off  CH4_output_duty=0.00  CH4_pulse=0
      settings: SourceProductName=Target Support Package - STM32 Adapter
  wires:
  Constant/1 -> GPIO_Write/1
  Constant1/1 -> GPIO_Write/2
  Product/1 -> Timers/1
  Data Store Read/1 -> Product/1
  Constant2/1 -> Product/2

== system BanlanceCar/Function-Call Subsystem/Subsystem6/If Action Subsystem3 ==
  Action Port : ActionPort  ActionPortLabel=if(u1 > 0)
  Constant4 : Constant
  Constant5 : Constant  Value=0
  Data Store Read1 : DataStoreRead  DataStoreName=motob  IndexOptions=Index vector (dialog)  Indices=1  OutputSizes=1
  GPIO_Write1 : GPIO_Lib/GPIO_Write  Port_name=GPIOA  Pin0=off  Toggle_Pin0=off  Pin1=off  Toggle_Pin1=off  Pin2=off  Toggle_Pin2=off  Pin3=off  Toggle_Pin3=off  Pin4=off  Toggle_Pin4=off  Pin5=off  Toggle_Pin5=off  Pin6=on  Toggle_Pin6=off  Pin7=on  Toggle_Pin7=off  Pin8=off  Toggle_Pin8=off  Pin9=off  Toggle_Pin9=off  Pin10=off  Toggle_Pin10=off  Pin11=off  Toggle_Pin11=off  Pin12=off  Toggle_Pin12=off  Pin13=off  Toggle_Pin13=off  Pin14=off  Toggle_Pin14=off  Pin15=off  Toggle_Pin15=off  PinList="GPIOA4  5  6  7GPIOB9  10GPIOD1  2"
      settings: SourceProductName=Target Support Package - STM32 Adapter
  Timers1 : TIMERS_Lib/Timers  currentTIM=TIM2  TIM_Name=TIM2  sysUsingTimer=off  TIM_APBClock=72000000  TIM_Set_Clk=off  TIM_Prescaler=0  TIM_Clock=72000000.00  Variable_frequency=off  TIM_Set_OutFreq=off  TIM_ARR=1  Output_frequency=72000000.00  Repetition_counter=0  TIM_Mode=Up  TIM_DMA=none  TIM_IRQ=on  TIM_IRQ_ONLY=off  TIM_UP=off  TIM_TRG=off  TIM_COM=off  TIM_BRK=off  NbTIM=4  CH1_enable=off  CH1N_enable=off  CH1_type=Unknown  CH1_DMA=off  CH1_int=off  CH1_edge=Rising  CH1_div=1  CH1_variable_duty=off  CH1_set_pulse=off  CH1_output_duty=0.00  CH1_pulse=0  CH2_enable=off  CH2N_enable=off  CH2_type=Unknown  CH2_DMA=off  CH2_int=off  CH2_edge=Rising  CH2_div=1  CH2_variable_duty=off  CH2_set_pulse=off  CH2_output_duty=0.00  CH2_pulse=0  CH3_enable=on  CH3N_enable=off  CH3_type=Output_PWM  CH3_DMA=off  CH3_int=off  CH3_edge=Rising  CH3_div=1  CH3_variable_duty=off  CH3_set_pulse=off  CH3_output_duty=49900.00  CH3_pulse=500-1  CH4_enable=on  CH4N_enable=off  CH4_type=Output_PWM  CH4_DMA=off  CH4_int=off  CH4_edge=Rising  CH4_div=1  CH4_variable_duty=on  CH4_set_pulse=off  CH4_output_duty=0.00  CH4_pulse=0
      settings: SourceProductName=Target Support Package - STM32 Adapter
  wires:
  Constant5/1 -> GPIO_Write1/2
  Data Store Read1/1 -> Timers1/1
  Constant4/1 -> GPIO_Write1/1

== system BanlanceCar/Function-Call Subsystem/Subsystem6/If Action Subsystem4 ==
  Action Port : ActionPort  ActionPortLabel=elseif(u1 == 0)
  Constant4 : Constant  Value=0
  Constant5 : Constant  Value=0
  Data Store Read1 : DataStoreRead  DataStoreName=motob  IndexOptions=Index vector (dialog)  Indices=1  OutputSizes=1
  GPIO_Write1 : GPIO_Lib/GPIO_Write  Port_name=GPIOA  Pin0=off  Toggle_Pin0=off  Pin1=off  Toggle_Pin1=off  Pin2=off  Toggle_Pin2=off  Pin3=off  Toggle_Pin3=off  Pin4=off  Toggle_Pin4=off  Pin5=off  Toggle_Pin5=off  Pin6=on  Toggle_Pin6=off  Pin7=on  Toggle_Pin7=off  Pin8=off  Toggle_Pin8=off  Pin9=off  Toggle_Pin9=off  Pin10=off  Toggle_Pin10=off  Pin11=off  Toggle_Pin11=off  Pin12=off  Toggle_Pin12=off  Pin13=off  Toggle_Pin13=off  Pin14=off  Toggle_Pin14=off  Pin15=off  Toggle_Pin15=off  PinList="GPIOA4  5  6  7GPIOB9  10GPIOD1  2"
      settings: SourceProductName=Target Support Package - STM32 Adapter
  Timers1 : TIMERS_Lib/Timers  currentTIM=TIM2  TIM_Name=TIM2  sysUsingTimer=off  TIM_APBClock=72000000  TIM_Set_Clk=off  TIM_Prescaler=0  TIM_Clock=72000000.00  Variable_frequency=off  TIM_Set_OutFreq=off  TIM_ARR=1  Output_frequency=72000000.00  Repetition_counter=0  TIM_Mode=Up  TIM_DMA=none  TIM_IRQ=on  TIM_IRQ_ONLY=off  TIM_UP=off  TIM_TRG=off  TIM_COM=off  TIM_BRK=off  NbTIM=4  CH1_enable=off  CH1N_enable=off  CH1_type=Unknown  CH1_DMA=off  CH1_int=off  CH1_edge=Rising  CH1_div=1  CH1_variable_duty=off  CH1_set_pulse=off  CH1_output_duty=0.00  CH1_pulse=0  CH2_enable=off  CH2N_enable=off  CH2_type=Unknown  CH2_DMA=off  CH2_int=off  CH2_edge=Rising  CH2_div=1  CH2_variable_duty=off  CH2_set_pulse=off  CH2_output_duty=0.00  CH2_pulse=0  CH3_enable=on  CH3N_enable=off  CH3_type=Output_PWM  CH3_DMA=off  CH3_int=off  CH3_edge=Rising  CH3_div=1  CH3_variable_duty=off  CH3_set_pulse=off  CH3_output_duty=49900.00  CH3_pulse=500-1  CH4_enable=on  CH4N_enable=off  CH4_type=Output_PWM  CH4_DMA=off  CH4_int=off  CH4_edge=Rising  CH4_div=1  CH4_variable_duty=on  CH4_set_pulse=off  CH4_output_duty=0.00  CH4_pulse=0
      settings: SourceProductName=Target Support Package - STM32 Adapter
  wires:
  Data Store Read1/1 -> Timers1/1
  Constant5/1 -> GPIO_Write1/2
  Constant4/1 -> GPIO_Write1/1

== system BanlanceCar/Function-Call Subsystem/Subsystem6/If Action Subsystem5 ==
  Action Port : ActionPort  ActionPortLabel=else
  Constant : Constant  Value=-1
  Constant4 : Constant  Value=0
  Constant5 : Constant
  Data Store Read1 : DataStoreRead  DataStoreName=motob  IndexOptions=Index vector (dialog)  Indices=1  OutputSizes=1
  GPIO_Write1 : GPIO_Lib/GPIO_Write  Port_name=GPIOA  Pin0=off  Toggle_Pin0=off  Pin1=off  Toggle_Pin1=off  Pin2=off  Toggle_Pin2=off  Pin3=off  Toggle_Pin3=off  Pin4=off  Toggle_Pin4=off  Pin5=off  Toggle_Pin5=off  Pin6=on  Toggle_Pin6=off  Pin7=on  Toggle_Pin7=off  Pin8=off  Toggle_Pin8=off  Pin9=off  Toggle_Pin9=off  Pin10=off  Toggle_Pin10=off  Pin11=off  Toggle_Pin11=off  Pin12=off  Toggle_Pin12=off  Pin13=off  Toggle_Pin13=off  Pin14=off  Toggle_Pin14=off  Pin15=off  Toggle_Pin15=off  PinList="GPIOA4  5  6  7GPIOB9  10GPIOD1  2"
      settings: SourceProductName=Target Support Package - STM32 Adapter
  Product : Product
  Timers1 : TIMERS_Lib/Timers  currentTIM=TIM2  TIM_Name=TIM2  sysUsingTimer=off  TIM_APBClock=72000000  TIM_Set_Clk=off  TIM_Prescaler=0  TIM_Clock=72000000.00  Variable_frequency=off  TIM_Set_OutFreq=off  TIM_ARR=1  Output_frequency=72000000.00  Repetition_counter=0  TIM_Mode=Up  TIM_DMA=none  TIM_IRQ=on  TIM_IRQ_ONLY=off  TIM_UP=off  TIM_TRG=off  TIM_COM=off  TIM_BRK=off  NbTIM=4  CH1_enable=off  CH1N_enable=off  CH1_type=Unknown  CH1_DMA=off  CH1_int=off  CH1_edge=Rising  CH1_div=1  CH1_variable_duty=off  CH1_set_pulse=off  CH1_output_duty=0.00  CH1_pulse=0  CH2_enable=off  CH2N_enable=off  CH2_type=Unknown  CH2_DMA=off  CH2_int=off  CH2_edge=Rising  CH2_div=1  CH2_variable_duty=off  CH2_set_pulse=off  CH2_output_duty=0.00  CH2_pulse=0  CH3_enable=on  CH3N_enable=off  CH3_type=Output_PWM  CH3_DMA=off  CH3_int=off  CH3_edge=Rising  CH3_div=1  CH3_variable_duty=off  CH3_set_pulse=off  CH3_output_duty=49900.00  CH3_pulse=500-1  CH4_enable=on  CH4N_enable=off  CH4_type=Output_PWM  CH4_DMA=off  CH4_int=off  CH4_edge=Rising  CH4_div=1  CH4_variable_duty=on  CH4_set_pulse=off  CH4_output_duty=0.00  CH4_pulse=0
      settings: SourceProductName=Target Support Package - STM32 Adapter
  wires:
  Constant5/1 -> GPIO_Write1/2
  Constant4/1 -> GPIO_Write1/1
  Data Store Read1/1 -> Product/1
  Constant/1 -> Product/2
  Product/1 -> Timers1/1

== matlab function BanlanceCar/Function-Call Subsystem1/MATLAB Function ==
  data: u1 input; NbChar output; u2 input; Buff output
function [NbChar, Buff] = convert(u1,u2)
if coder.target('Sfun')
% Executing in MATLAB, Buff is null
Buff = uint32(0);
NbChar = uint16(0);
else
Buff = uint32(0);
string = char(zeros(1,31));
stringSize = uint16(size(string,2));
stringFormat = char(['u1= %7.0f,u2= %7.1f r/s',13,10,0]);
coder.ceval('snprintf',coder.wref(string),stringSize,coder.rref(stringFormat),u1,u2);
Buff = coder.ceval('getBuffPtr',coder.rref(string));
NbChar = stringSize;
end
end
